simulink model "ThdRwLtStBkReclnCtrl"  (R2024b)
settings: Solver=FixedStepDiscrete  StartTime=0.0  StopTime=10.0  FixedStep=0.01  RelTol=1e-3
undefined symbols (not defined in the file or in its folder): KeSMSuMdMotFinshdTm_Val, KeSMSuMdRetryTm1_Val, KeSMSuModeReqDurgTm_Val, KeSMSwThdRwLtStBkReclnEnTrigBitMask6s_Val, KeSMSwThdRwLtStBkReclnEnTrigBitMask_Val
libraries: StCtrlLib x1
settings Model: ModifiedHistory=24.1.2  Creator=sn2xws  LastModifiedBy=sn55gm
settings SolverCC: AlgebraicLoopSolver=TrustRegion
settings DataIOCC: SaveFormat=StructureWithTime  ReturnWorkspaceOutputs=off
settings OptimizationCC: DefaultParameterBehavior=Inlined  EnhancedBackFolding=on  PassReuseOutputArgsAs=Individual arguments  ZeroExternalMemoryAtStartup=off  ZeroInternalMemoryAtStartup=off  OptimizeBlockOrder=speed  DifferentSizesBufferReuse=on  OptimizationCustomize=off  EfficientTunableParamExpr=on
settings DebuggingCC: SignalInfNanChecking=error  ParameterTunabilityLossMsg=error  UnconnectedInputMsg=warning  UnconnectedOutputMsg=warning  UnconnectedLineMsg=warning  AssertControl=DisableAll  SFUndirectedBroadcastEventsDiag=error  ArithmeticOperatorsInVariantConditions=warning
settings ModelReferenceCC: EnableRefExpFcnMdlSchedulingChecks=on  ModelReferenceNumInstancesAllowed=Single
settings SFSimCC: CompileTimeRecursionLimit=0  EnableRuntimeRecursion=off  MATLABDynamicMemAlloc=off  CustomCodeUndefinedFunction=UseInterfaceOnly
settings RTWCC: Description=AUTOSAR  SystemTargetFile=autosar.tlc  GenCodeOnly=on  TemplateMakefile=ert_default_tmf  GenerateReport=on  IncludeHyperlinkInReport=on  LaunchReport=on  DataTypeReplacement=CDataTypesFixedWidth  GenerateTraceInfo=on  GenerateTraceReport=on  GenerateTraceReportSl=on  GenerateTraceReportSf=on  GenerateTraceReportEml=on  GPUComputeCapability=3.5
settings CodeAppCC: ForceParamTrailComments=on  IgnoreCustomStorageClasses=off  OperatorAnnotations=on  SimulinkDataObjDesc=on  SFDataObjDesc=on  InsertBlockDesc=on
settings STFCustomTargetCC: TargetLangStandard=C99 (ISO)  UtilityFuncGeneration=Shared location  MultiwordLength=256  ParMdlRefBuildCompliant=on  CompOptLevelCompliant=on  IncludeMdlTerminateFcn=off  CombineOutputUpdateFcns=on  SuppressErrorStatus=on  ERTCustomFileBanners=on  SupportNonFinite=off  SupportComplex=off  SupportContinuousTime=off  SupportNonInlinedSFcns=off  RemoveResetFunc=on  ParenthesesLevel=Maximum  CastingMode=Standards  MATLABClassNameForMDSCustomization=Simulink.SoftwareTarget.ERTCustomization  AutosarCompliant=on  UseToolchainInfoCompliant=on  LookupTableObjectStructAxisOrder=2,1,3,4,...  LUTObjectStructOrderEvenSpacing=Size,Table,Breakpoints  SystemTargetFile=autosar.tlc
settings ERTTargetCC: TargetLangStandard=C99 (ISO)  UtilityFuncGeneration=Shared location  ConcurrentExecutionCompliant=off  IncludeMdlTerminateFcn=off  SuppressErrorStatus=on  SupportNonFinite=off  SupportComplex=off  ParenthesesLevel=Maximum  CastingMode=Standards  ModelStepFunctionPrototypeControlCompliant=off  CPPClassGenCompliant=off  AutosarCompliant=on  LookupTableObjectStructAxisOrder=2,1,3,4,...  LUTObjectStructOrderEvenSpacing=Size,Table,Breakpoints  ERTCustomFileTemplate=example_file_process.tlc  ERTFilePackagingFormat=Compact  EnableSignedLeftShifts=off  EnableSignedRightShifts=off  BooleanTrueId=TRUE  BooleanFalseId=FALSE  DynamicArrayContainerType=coder::array

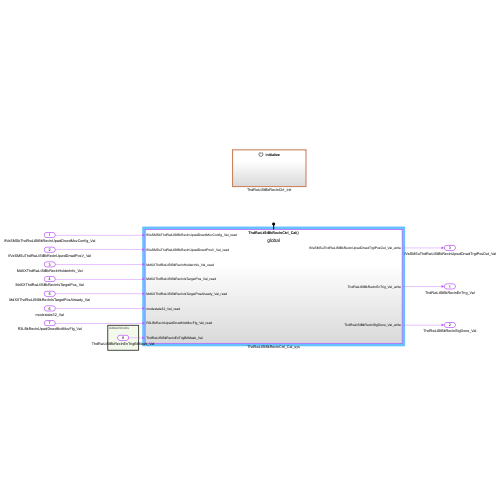
[thumbnail: Simulink's stored preview of the top-level diagram]
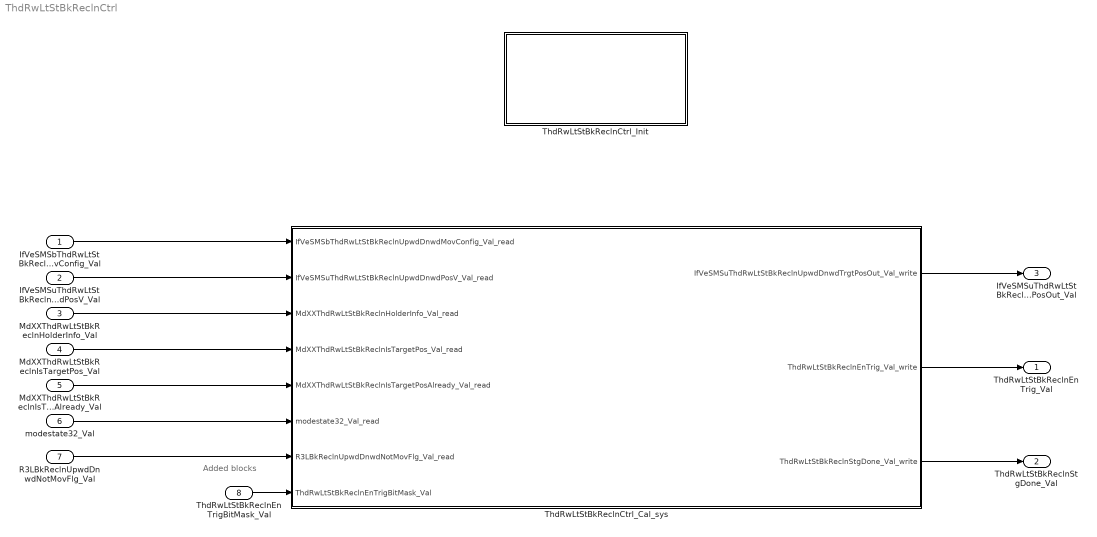
== system ThdRwLtStBkReclnCtrl ==
  note: Added blocks
  IfVeSMSbThdRwLtStBkReclnUpwdDnwdMovConfig_Val : Inport  OutDataTypeStr=boolean  PortDimensions=1
  IfVeSMSuThdRwLtStBkReclnUpwdDnwdPosV_Val : Inport  Port=2  OutDataTypeStr=boolean  PortDimensions=1
  MdXXThdRwLtStBkReclnHolderInfo_Val : Inport  Port=3  OutDataTypeStr=uint32  PortDimensions=1
  MdXXThdRwLtStBkReclnIsTargetPos_Val : Inport  Port=4  OutDataTypeStr=uint32  PortDimensions=1
  MdXXThdRwLtStBkReclnIsTargetPosAlready_Val : Inport  Port=5  OutDataTypeStr=uint32  PortDimensions=1
  modestate32_Val : Inport  Port=6  OutDataTypeStr=uint32  PortDimensions=1
  R3LBkReclnUpwdDnwdNotMovFlg_Val : Inport  Port=7  OutDataTypeStr=boolean  PortDimensions=1
  ThdRwLtStBkReclnEnTrigBitMask_Val : Inport  Port=8  OutDataTypeStr=uint32  PortDimensions=1
  ThdRwLtStBkReclnCtrl_Cal_sys : Subsystem
  ThdRwLtStBkReclnCtrl_Init : Subsystem
  ThdRwLtStBkReclnEnTrig_Val : Outport  OutDataTypeStr=boolean  PortDimensions=1  VectorParamsAs1DForOutWhenUnconnected=off
  ThdRwLtStBkReclnStgDone_Val : Outport  Port=2  OutDataTypeStr=boolean  PortDimensions=1  VectorParamsAs1DForOutWhenUnconnected=off
  IfVeSMSuThdRwLtStBkReclnUpwdDnwdTrgtPosOut_Val : Outport  Port=3  OutDataTypeStr=boolean  PortDimensions=1  VectorParamsAs1DForOutWhenUnconnected=off
  wires:
  IfVeSMSbThdRwLtStBkReclnUpwdDnwdMovConfig_Val/1 -> ThdRwLtStBkReclnCtrl_Cal_sys/1(IfVeSMSbThdRwLtStBkReclnUpwdDnwdMovConfig_Val_read)
  IfVeSMSuThdRwLtStBkReclnUpwdDnwdPosV_Val/1 -> ThdRwLtStBkReclnCtrl_Cal_sys/2(IfVeSMSuThdRwLtStBkReclnUpwdDnwdPosV_Val_read)
  MdXXThdRwLtStBkReclnHolderInfo_Val/1 -> ThdRwLtStBkReclnCtrl_Cal_sys/3(MdXXThdRwLtStBkReclnHolderInfo_Val_read)
  MdXXThdRwLtStBkReclnIsTargetPos_Val/1 -> ThdRwLtStBkReclnCtrl_Cal_sys/4(MdXXThdRwLtStBkReclnIsTargetPos_Val_read)
  MdXXThdRwLtStBkReclnIsTargetPosAlready_Val/1 -> ThdRwLtStBkReclnCtrl_Cal_sys/5(MdXXThdRwLtStBkReclnIsTargetPosAlready_Val_read)
  modestate32_Val/1 -> ThdRwLtStBkReclnCtrl_Cal_sys/6(modestate32_Val_read)
  R3LBkReclnUpwdDnwdNotMovFlg_Val/1 -> ThdRwLtStBkReclnCtrl_Cal_sys/7(R3LBkReclnUpwdDnwdNotMovFlg_Val_read)
  ThdRwLtStBkReclnCtrl_Cal_sys/1(IfVeSMSuThdRwLtStBkReclnUpwdDnwdTrgtPosOut_Val_write) -> IfVeSMSuThdRwLtStBkReclnUpwdDnwdTrgtPosOut_Val/1
  ThdRwLtStBkReclnCtrl_Cal_sys/2(ThdRwLtStBkReclnEnTrig_Val_write) -> ThdRwLtStBkReclnEnTrig_Val/1
  ThdRwLtStBkReclnCtrl_Cal_sys/3(ThdRwLtStBkReclnStgDone_Val_write) -> ThdRwLtStBkReclnStgDone_Val/1
  ThdRwLtStBkReclnEnTrigBitMask_Val/1 -> ThdRwLtStBkReclnCtrl_Cal_sys/8(ThdRwLtStBkReclnEnTrigBitMask_Val)

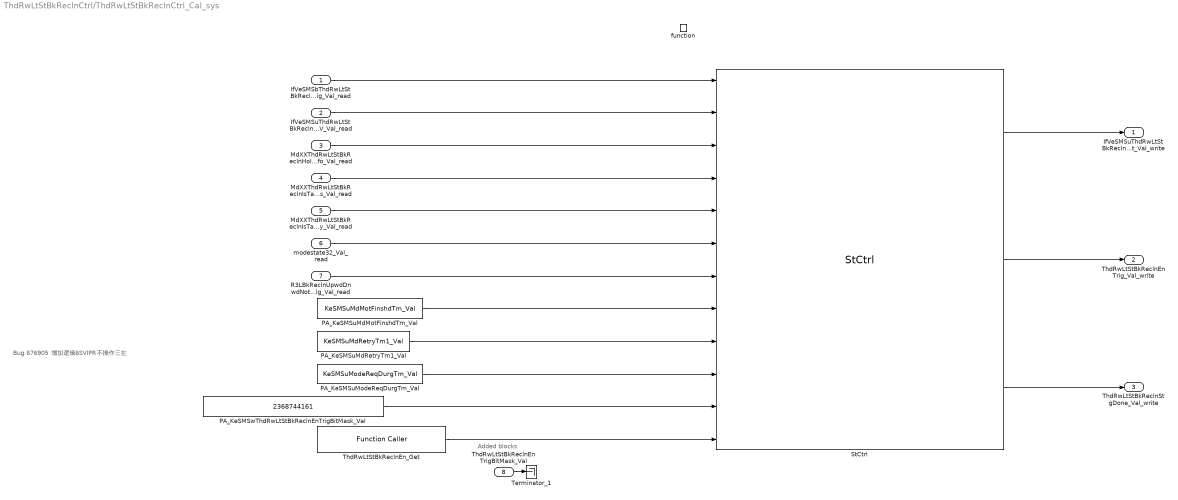
== system ThdRwLtStBkReclnCtrl/ThdRwLtStBkReclnCtrl_Cal_sys ==
  note: Bug 676905 增加逻辑6SVIPR不操作三左
  note: Added blocks
  IfVeSMSbThdRwLtStBkReclnUpwdDnwdMovConfig_Val_read : Inport
  IfVeSMSuThdRwLtStBkReclnUpwdDnwdPosV_Val_read : Inport  Port=2
  MdXXThdRwLtStBkReclnHolderInfo_Val_read : Inport  Port=3
  MdXXThdRwLtStBkReclnIsTargetPos_Val_read : Inport  Port=4
  MdXXThdRwLtStBkReclnIsTargetPosAlready_Val_read : Inport  Port=5
  modestate32_Val_read : Inport  Port=6
  R3LBkReclnUpwdDnwdNotMovFlg_Val_read : Inport  Port=7
  ThdRwLtStBkReclnEnTrigBitMask_Val : Inport  Port=8
  function : TriggerPort  TriggerType=function-call  IsSimulinkFunction=on  FunctionName=ThdRwLtStBkReclnCtrl_Cal  VariantControl=(inherit)
  PA_KeSMSuMdMotFinshdTm_Val : Constant  Value=KeSMSuMdMotFinshdTm_Val
  PA_KeSMSuMdRetryTm1_Val : Constant  Value=KeSMSuMdRetryTm1_Val
  PA_KeSMSuModeReqDurgTm_Val : Constant  Value=KeSMSuModeReqDurgTm_Val
  PA_KeSMSwThdRwLtStBkReclnEnTrigBitMask_Val : Constant  Value=2368744161  OutDataTypeStr=uint32
  StCtrl : StCtrlLib/StCtrl  SystemSampleTime=-1  VariantActivationTime=update diagram  AllowFlexibleInterface=on  Latency=0  AutoFrameSizeCalculation=off
  Terminator_1 : Terminator
  ThdRwLtStBkReclnEn_Get : FunctionCaller  FunctionPrototype=data = ThdRwLtStBkReclnEn_Get()  InputArgumentSpecifications=<Enter example>  OutputArgumentSpecifications=uint32(1)
  IfVeSMSuThdRwLtStBkReclnUpwdDnwdTrgtPosOut_Val_write : Outport  VectorParamsAs1DForOutWhenUnconnected=off
      settings: EnsureOutportIsVirtual=on
  ThdRwLtStBkReclnEnTrig_Val_write : Outport  Port=2  VectorParamsAs1DForOutWhenUnconnected=off
      settings: EnsureOutportIsVirtual=on
  ThdRwLtStBkReclnStgDone_Val_write : Outport  Port=3  VectorParamsAs1DForOutWhenUnconnected=off
      settings: EnsureOutportIsVirtual=on
  wires:
  StCtrl/1 -> IfVeSMSuThdRwLtStBkReclnUpwdDnwdTrgtPosOut_Val_write/1
  StCtrl/2 -> ThdRwLtStBkReclnEnTrig_Val_write/1
  StCtrl/3 -> ThdRwLtStBkReclnStgDone_Val_write/1
  IfVeSMSbThdRwLtStBkReclnUpwdDnwdMovConfig_Val_read/1 -> StCtrl/1
  IfVeSMSuThdRwLtStBkReclnUpwdDnwdPosV_Val_read/1 -> StCtrl/2
  MdXXThdRwLtStBkReclnHolderInfo_Val_read/1 -> StCtrl/3
  MdXXThdRwLtStBkReclnIsTargetPos_Val_read/1 -> StCtrl/4
  MdXXThdRwLtStBkReclnIsTargetPosAlready_Val_read/1 -> StCtrl/5
  modestate32_Val_read/1 -> StCtrl/6
  R3LBkReclnUpwdDnwdNotMovFlg_Val_read/1 -> StCtrl/7
  ThdRwLtStBkReclnEn_Get/1 -> StCtrl/12
  PA_KeSMSuModeReqDurgTm_Val/1 -> StCtrl/10
  PA_KeSMSuMdRetryTm1_Val/1 -> StCtrl/9
  PA_KeSMSuMdMotFinshdTm_Val/1 -> StCtrl/8
  PA_KeSMSwThdRwLtStBkReclnEnTrigBitMask_Val/1 -> StCtrl/11
  ThdRwLtStBkReclnEnTrigBitMask_Val/1 -> Terminator_1/1

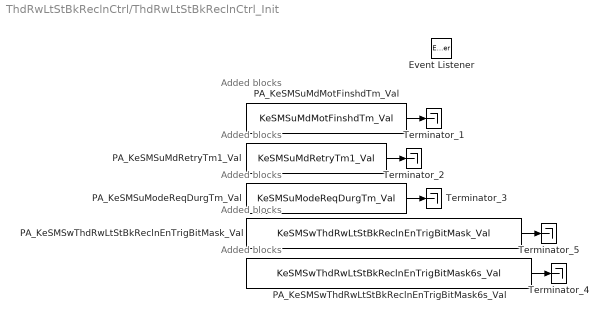
== system ThdRwLtStBkReclnCtrl/ThdRwLtStBkReclnCtrl_Init ==
  note: Added blocks
  note: Added blocks
  note: Added blocks
  note: Added blocks
  note: Added blocks
  Event Listener : EventListener  EventName=reset
  PA_KeSMSuMdMotFinshdTm_Val : Constant  Value=KeSMSuMdMotFinshdTm_Val
  PA_KeSMSuMdRetryTm1_Val : Constant  Value=KeSMSuMdRetryTm1_Val
  PA_KeSMSuModeReqDurgTm_Val : Constant  Value=KeSMSuModeReqDurgTm_Val
  PA_KeSMSwThdRwLtStBkReclnEnTrigBitMask6s_Val : Constant  Value=KeSMSwThdRwLtStBkReclnEnTrigBitMask6s_Val
  PA_KeSMSwThdRwLtStBkReclnEnTrigBitMask_Val : Constant  Value=KeSMSwThdRwLtStBkReclnEnTrigBitMask_Val
  Terminator_{1..5} (5 alike) : Terminator
  wires:
  PA_KeSMSuMdMotFinshdTm_Val/1 -> Terminator_1/1
  PA_KeSMSuMdRetryTm1_Val/1 -> Terminator_2/1
  PA_KeSMSuModeReqDurgTm_Val/1 -> Terminator_3/1
  PA_KeSMSwThdRwLtStBkReclnEnTrigBitMask6s_Val/1 -> Terminator_4/1
  PA_KeSMSwThdRwLtStBkReclnEnTrigBitMask_Val/1 -> Terminator_5/1
